simulink library "INT_EngPrt_TrqLimCalc"  (R2016b)
settings: Solver=VariableStepAuto  StartTime=0.0  StopTime=10.0  RelTol=1e-3
settings Model: Creator=lenovo  LastModifiedBy=lenovo

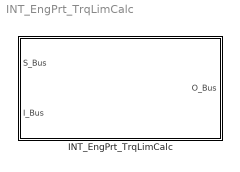
== system INT_EngPrt_TrqLimCalc ==
  INT_EngPrt_TrqLimCalc : Subsystem

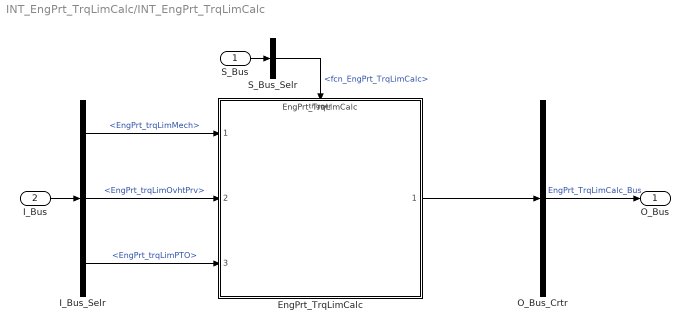
== system INT_EngPrt_TrqLimCalc/INT_EngPrt_TrqLimCalc ==
  S_Bus : Inport
  I_Bus : Inport  Port=2
  EngPrt_TrqLimCalc : ModelReference  ModelNameDialog=EngPrt_TrqLimCalc  SimulationMode=Normal  ModelReferenceVersion=1.5  TriggerPortName=function  TriggerPortTriggerType=function-call  TriggerPortStatesWhenEnabling=held
  I_Bus_Selr : BusSelector  OutputSignals=EngPrt_trqLimMech,EngPrt_trqLimOvhtPrv,EngPrt_trqLimPTO
  O_Bus_Crtr : BusCreator  Inputs=1
  S_Bus_Selr : BusSelector  OutputSignals=fcn_EngPrt_TrqLimCalc
  O_Bus : Outport
  wires:
  S_Bus_Selr/1 -> EngPrt_TrqLimCalc/Trigger  "<fcn_EngPrt_TrqLimCalc>"
  S_Bus/1 -> S_Bus_Selr/1
  I_Bus/1 -> I_Bus_Selr/1
  I_Bus_Selr/1 -> EngPrt_TrqLimCalc/1  "<EngPrt_trqLimMech>"
  I_Bus_Selr/2 -> EngPrt_TrqLimCalc/2  "<EngPrt_trqLimOvhtPrv>"
  I_Bus_Selr/3 -> EngPrt_TrqLimCalc/3  "<EngPrt_trqLimPTO>"
  O_Bus_Crtr/1 -> O_Bus/1  "EngPrt_TrqLimCalc_Bus"
  EngPrt_TrqLimCalc/1 -> O_Bus_Crtr/1
